simulink model "sixDOF"  (R2020b)
settings: Solver=VariableStepAuto  StartTime=0.0  StopTime=50  RelTol=1e-3
values from neighbouring files (symbols this model uses):
  A_AD = horzcat(A_i, A_ii)    [six.m]
  A_kal = [0 0 0 1 0 0 ... (first row only)    [six.m]
  B_AD = horzcat(B_i, B_ii)    [six.m]
  B_kal = [0 0 0 0 0 0 ... (first row only)    [six.m]
  C_AD = eye(6)    [six.m]
  C_D = 0.2    [Point_Mass.m]    (also in Point_mass_fancy_results.m = 0.6; point_mass_MAIN.m = 0.02; point_mass_unit_test_func.m = C_D; point_mass_verification.m)
  C_kal = eye(6)    [six.m]
  D_AD = zeros(6)    [six.m]
  D_kal = zeros(6)    [six.m]
  g = theta_dd_0*theta_d_0*cos(theta_0)*I_xy - phi_d_0*(theta_d_0)^2*sin(theta_0)*I_xy - phi_dd_0*theta_d_0*sin(theta_0)*I_xz - theta_d_0^2 * cos(theta_0)*I_xz + phi_d_0 * I_zx * theta_d_0 * cos(theta_0) + I_zy*phi_d_0^2*theta_d_0*sin(2*theta_0) + I_zz*phi_d_0 * theta_d_0 * cos(2*theta_0) + phi_d_0 * theta_d_0 * I_yx * sin(theta_0) - phi_d_0^2 * I_yy * theta_d_0 * cos(2*theta_0) + phi_d_0^2 * theta_d_0  ...(+23 chars)    [Gyro.m]    (also in Point_Mass.m = 9.81; Point_mass_fancy_results.m = 9.81; Tdt.m = cos(phi)*sin(theta)*cos(psi) + sin(phi)*sin(psi); angular_tune.m = (I_yx*I_zy - I_yy*I_zx)*(I_zx*wy_0 - I_yx*wz_0) + (I_xy*I_zx)
  I_inv = diag(I_mat)    [Propellers_tilt.m]    (also in six.m = Inertia_inv; tilt_verification.m = I_inv*0)
  I_mat = I_diag    [Propellers_tilt.m]    (also in six.m = Inertia; tilt_verification.m = 0)
  m = theta_d_0*cos(theta_0)*I_yy - theta_d_0*sin(theta_0)*I_yz + I_xx*cos(theta_0)*theta_d_0 + 2*phi_d_0*I_xy*cos(theta_0)*sin(theta_0) + 2*phi_d_0*I_xz*(cos(theta_0))^2 - theta_d_0 * I_zy * sin(theta_0) - theta_d_0*cos(theta_0)*I_zz    [Gyro.m]    (also in Point_Mass.m = 100; Point_mass_fancy_results.m = 600; point_mass_MAIN.m = 640; point_mass_unit_test_func.m = mass)
  rho = 0.991    [Point_Mass.m]    (also in Point_mass_fancy_results.m = 1.225; point_mass_MAIN.m = 1.225; point_mass_unit_test_func.m = density; point_mass_verification.m = 1.225)
  S = 4.5    [Point_Mass.m]    (also in Point_mass_fancy_results.m = 1.8; point_mass_MAIN.m = 2; point_mass_unit_test_func.m = S; point_mass_verification.m = 2)
  T = 10.5    [Point_mass_fancy_results.m]    (also in point_mass_MAIN.m; point_mass_unit_test_func.m = T; point_mass_verification.m = 1.5; six.m)
  time_delay = 0.3    [Point_mass_fancy_results.m]    (also in point_mass_MAIN.m = 3e-05; point_mass_unit_test_func.m = time_delay; point_mass_verification.m = 0.1; six.m = 0.1)
undefined symbols (not defined in the file or in its folder): Continuous, Time
libraries: pid_lib x6, ctrlSharedLib x2, simulink x2, sharedutil x1
settings Model: Creator=Jonathan van Zyl  LastModifiedBy=Jonathan van Zyl

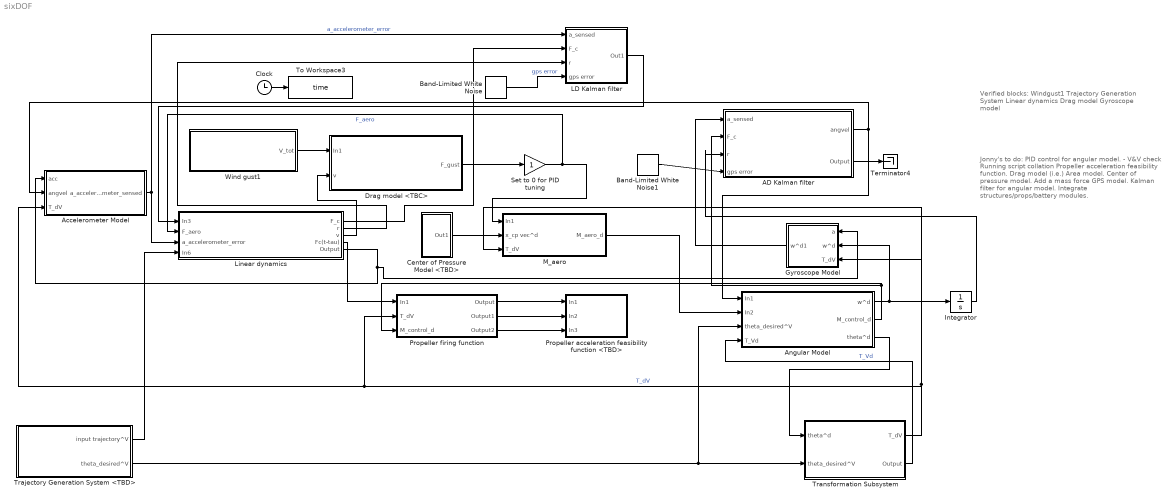
== system sixDOF ==
  note: Jonny's to do:
      | PID control for angular model. - V&V check
      | Running script collation
      | Propeller acceleration feasibility function.
      | Drag model (i.e.) Area model.
      | Center of pressure model.
      | Add a mass force
      | GPS model.
      | Kalman filter for angular model.
      | Integrate structures/props/battery modules.
  note: Verified blocks:
      | Windgust1
      | Trajectory Generation System
      | Linear dynamics
      | Drag model
      | Gyroscope model
  AD Kalman filter : Subsystem
  Accelerometer Model : Subsystem
  Angular Model : Subsystem
  Band-Limited White Noise : simulink/Sources/Band-Limited White Noise  Cov=[0.01]  Ts=0.1  seed=[23341]
  Band-Limited White Noise1 : simulink/Sources/Band-Limited White Noise  Cov=[0.01]  Ts=0.1  seed=[23341]
  Center of Pressure Model <TBD> : Subsystem
  Clock : Clock
  Drag model <TBC> : Subsystem
  Gyroscope Model : Subsystem
  Integrator : Integrator  InitialCondition=[0;0;0]
  LD Kalman filter : Subsystem
  Linear dynamics : Subsystem
  M_aero : Subsystem
  Propeller acceleration feasibility function <TBD> : Subsystem
  Propeller firing function : Subsystem
  Set to 0 for PID tuning : Gain
  Terminator4 : Terminator
  To Workspace3 : ToWorkspace  VariableName=time  SaveFormat=Structure  SampleTime=-1
      settings: Save2DSignal=2-D array (concatenate along first dimension)
  Trajectory Generation System <TBD> : Subsystem
  Transformation Subsystem : Subsystem
  Wind gust1 : Subsystem
  wires:
  Clock/1 -> To Workspace3/1
  Wind gust1/1(V_tot) -> Drag model <TBC>/1(In1)
  Drag model <TBC>/1(F_gust) -> Set to 0 for PID tuning/1
  Transformation Subsystem/1(T_dV) -> Gyroscope Model/3(T_dV), Accelerometer Model/3(T_dV), Propeller firing function/2(T_dV), M_aero/3(T_dV)  "T_dV"
  Center of Pressure Model <TBD>/1(Out1) -> M_aero/2(x_cp vec^d)
  M_aero/1(M_aero_d) -> Angular Model/2(In2)
  Transformation Subsystem/2(Output) -> Angular Model/4(T_Vd)  "T_Vd"
  Angular Model/1(w^d) -> Integrator/1, Gyroscope Model/2(w^d)
  Angular Model/2(M_control_d) -> AD Kalman filter/2(F_c), Propeller firing function/3(M_control_d)
  Angular Model/3(theta^d) -> Transformation Subsystem/1(theta^d)
  Trajectory Generation System <TBD>/2(theta_desired^V) -> Transformation Subsystem/2(theta_desired^V), Angular Model/3(theta_desired^V)
  Propeller firing function/1(Output) -> Propeller acceleration feasibility function <TBD>/1(In1)
  Propeller firing function/2(Output1) -> Propeller acceleration feasibility function <TBD>/2(In2)
  Propeller firing function/3(Output2) -> Propeller acceleration feasibility function <TBD>/3(In3)
  Band-Limited White Noise/1 -> LD Kalman filter/4(gps error)  "gps error"
  Set to 0 for PID tuning/1 -> Linear dynamics/2(F_aero), M_aero/1(In1)  "F_aero"
  Linear dynamics/5(Output) -> Gyroscope Model/1(a), Accelerometer Model/1(acc)
  LD Kalman filter/1(Out1) -> Linear dynamics/1(In3)
  Accelerometer Model/1(a_accelerometer_sensed) -> Linear dynamics/3(a_accelerometer_error), LD Kalman filter/1(a_sensed)  "a_accelerometer_error"
  Trajectory Generation System <TBD>/1(input trajectory^V) -> Linear dynamics/4(In6)
  Linear dynamics/1(F_c) -> LD Kalman filter/2(F_c)
  Linear dynamics/2(r) -> LD Kalman filter/3(r)
  Linear dynamics/3(v) -> Drag model <TBC>/2(v)
  Linear dynamics/4(Fc(t-tau)) -> Propeller firing function/1(In1)
  AD Kalman filter/1(angvel) -> Angular Model/1(In1), Accelerometer Model/2(angvel)
  Gyroscope Model/1(w^d1) -> AD Kalman filter/1(a_sensed)
  AD Kalman filter/2(Output) -> Terminator4/1
  Integrator/1 -> AD Kalman filter/3(r)
  Band-Limited White Noise1/1 -> AD Kalman filter/4(gps error)

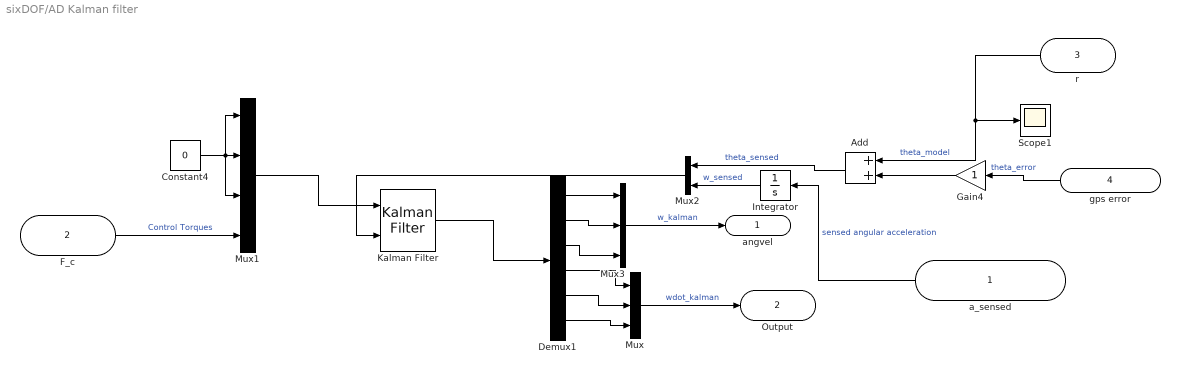
== system sixDOF/AD Kalman filter ==
  a_sensed : Inport
  F_c : Inport  Port=2
  r : Inport  Port=3
  gps error : Inport  Port=4
  Add : Sum
  Constant4 : Constant  Value=0
  Demux1 : Demux  Outputs=6
  Gain4 : Gain
  Integrator : Integrator  InitialCondition=[0;0;0]
  Kalman Filter : ctrlSharedLib/Kalman Filter  TimeDomain=Continuous-Time  UseCurrentEstimator=on  ModelSource=Individual A, B, C, D matrices  ModelSourceVariable=ss(0.95,1,1,0,1)  A=A_AD  B=B_AD  C=C_AD  D=D_AD  NumberOfStates=1  NumberOfInputs=1  NumberOfOutputs=1  InitialEstimateSource=Dialog  X0=[0;0;0;0;0;0]  P0=10  UseK=off  UseGH=off  NumberOfProcessNoiseInputs=1  G=1  TimeInvariantG=on  H=0  TimeInvariantH=on  Q=0.05  TimeInvariantQ=on  R=1  TimeInvariantR=on  N=0  TimeInvariantN=on  AddInputPort=on  AddEnablePort=off  OutputEstimatedY=off  OutputP=off  Ts=-1
  Mux : Mux  Inputs=3
  Mux1 : Mux
  Mux2 : Mux  Inputs=2
  Mux3 : Mux  Inputs=3
  Scope1 : Scope
  angvel : Outport
  Output : Outport  Port=2
  wires:
  Demux1/5 -> Mux/2
  Mux2/1 -> Kalman Filter/2
  Constant4/1 -> Mux1/3, Mux1/1, Mux1/2
  gps error/1 -> Gain4/1  "theta_error"
  r/1 -> Scope1/1, Add/1  "theta_model"
  Demux1/4 -> Mux/1
  Demux1/2 -> Mux3/2
  Mux1/1 -> Kalman Filter/1
  F_c/1 -> Mux1/4  "Control Torques"
  Demux1/1 -> Mux3/1
  Kalman Filter/1 -> Demux1/1
  Demux1/6 -> Mux/3
  Gain4/1 -> Add/2
  Demux1/3 -> Mux3/3
  Integrator/1 -> Mux2/2  "w_sensed"
  Add/1 -> Mux2/1  "theta_sensed"
  Mux3/1 -> angvel/1  "w_kalman"
  a_sensed/1 -> Integrator/1  "sensed angular acceleration"
  Mux/1 -> Output/1  "wdot_kalman"

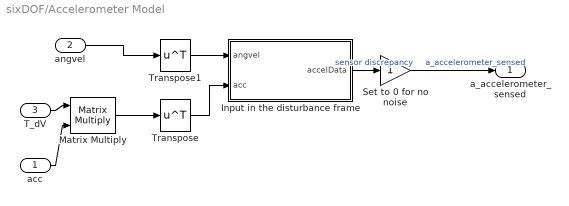
== system sixDOF/Accelerometer Model ==
  acc : Inport
  angvel : Inport  Port=2
  T_dV : Inport  Port=3
  Input in the disturbance frame : MATLAB Function  TreatAsAtomicUnit=on
  Matrix Multiply : Product  Multiplication=Matrix(*)
  Set to 0 for no noise : Gain
  Transpose : Math  Operator=transpose  SaturateOnIntegerOverflow=on
  Transpose1 : Math  Operator=transpose  SaturateOnIntegerOverflow=on
  a_accelerometer_sensed : Outport
  wires:
  Input in the disturbance frame/1(accelData) -> Set to 0 for no noise/1  "sensor discrepancy"
  acc/1 -> Matrix Multiply/2
  angvel/1 -> Transpose1/1
  Set to 0 for no noise/1 -> a_accelerometer_sensed/1  "a_accelerometer_sensed"
  Matrix Multiply/1 -> Transpose/1
  T_dV/1 -> Matrix Multiply/1
  Transpose/1 -> Input in the disturbance frame/2(acc)
  Transpose1/1 -> Input in the disturbance frame/1(angvel)

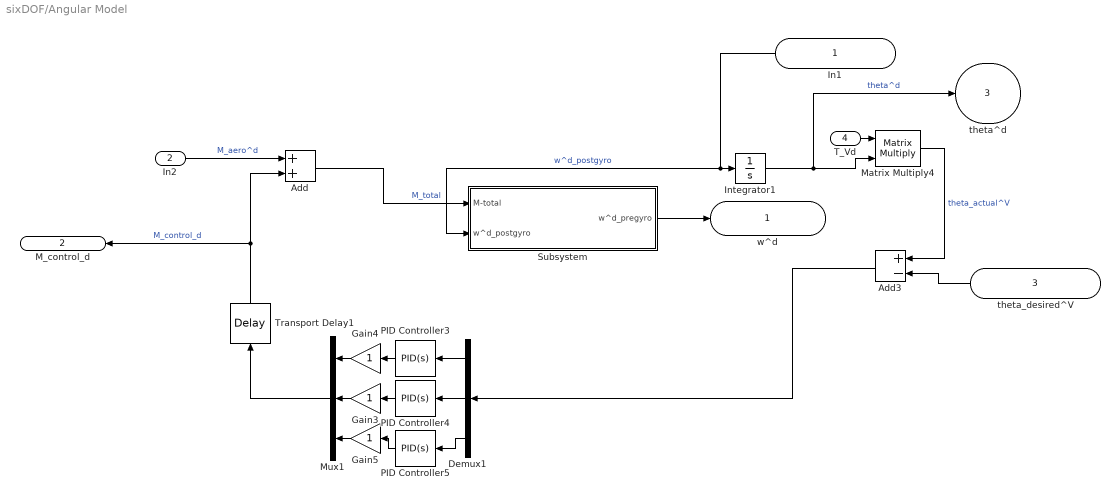
== system sixDOF/Angular Model ==
  In1 : Inport
  In2 : Inport  Port=2
  theta_desired^V : Inport  Port=3
  T_Vd : Inport  Port=4
  Add : Sum
  Add3 : Sum  Inputs=+-
  Demux1 : Demux  Outputs=3
  Gain3 : Gain
  Gain4 : Gain
  Gain5 : Gain
  Integrator1 : Integrator  InitialCondition=[0;0;0]
  Matrix Multiply4 : Product  Multiplication=Matrix(*)
  Mux1 : Mux  Inputs=3
  PID Controller3 : pid_lib/PID Controller  Controller=PID  Form=Parallel  TimeDomain=Continuous-time  UseExternalTs=off  SampleTime=-1  IntegratorMethod=Forward Euler  FilterMethod=Forward Euler  ControllerParametersSource=internal  P=1  I=1  D=0  UseFilter=on  N=100  TunerSelectOption=Transfer Function Based (PID Tuner App)  InitialConditionSource=internal  InitialConditionForIntegrator=0  InitialConditionForFilter=0  DifferentiatorICPrevScaledInput=0  ExternalReset=none  TrackingMode=off  Kt=1  LimitOutput=off  SatLimitsSource=internal  UpperSaturationLimit=inf  LowerSaturationLimit=-inf  LinearizeAsGain=on  AntiWindupMode=none  Kb=1  POutMin=[]  POutMax=[]  IOutMin=[]  IOutMax=[]  DOutMin=[]  DOutMax=[]  NOutMin=[]  NOutMax=[]  SumOutMin=[]  SumOutMax=[]  SaturationOutMin=[]  SaturationOutMax=[]  PParamMin=[]  PParamMax=[]  IParamMin=[]  IParamMax=[]  DParamMin=[]  DParamMax=[]  NParamMin=[]  NParamMax=[]  KbParamMin=[]  KbParamMax=[]  KtParamMin=[]  KtParamMax=[]  KbOutMin=[]  KbOutMax=[]  KtOutMin=[]  KtOutMax=[]  IntegratorOutMin=[]  IntegratorOutMax=[]  FilterOutMin=[]  FilterOutMax=[]  SumI1OutMin=[]  SumI1OutMax=[]  SumI2OutMin=[]  SumI2OutMax=[]  SumI3OutMin=[]  SumI3OutMax=[]  SumI4OutMin=[]  SumI4OutMax=[]  SumDOutMin=[]  SumDOutMax=[]  DifferentiatorOutMin=[]  DifferentiatorOutMax=[]  FilterDiffOutCoefMin=[]  FilterDiffOutCoefMax=[]  ReciprocalOutMin=[]  ReciprocalOutMax=[]  SumDenOutMin=[]  SumDenOutMax=[]  SumNumOutMin=[]  SumNumOutMax=[]  DivideOutMin=[]  DivideOutMax=[]  UdiffTsProdOutMin=[]  UdiffTsProdOutMax=[]  NTsProdOutMin=[]  NTsProdOutMax=[]  UintegralTsProdOutMin=[]  UintegralTsProdOutMax=[]  UngainTsProdOutMin=[]  UngainTsProdOutMax=[]  IntegratorContinuousStateAttributes=''  IntegratorStateMustResolveToSignalObject=off  IntegratorRTWStateStorageClass=Auto  FilterContinuousStateAttributes=''  FilterStateMustResolveToSignalObject=off  FilterRTWStateStorageClass=Auto  ParallelPVariant=InternalParameters  IdealPVariant=Disabled  IVariant=InternalParameters  DVariant=InternalParameters  IntegratorVariant=Continuous  SatVariant=Disabled  AWVariant=Passthrough  PCopyVariant=Disabled  TRVariant=Disabled  FdbkBlocksVariant=Forward  IdealPFdbkVariant=Disabled  SatFdbkVariant=Disabled  DerivativeFilterVariant=ContFilter  NVariant=InternalParameters  NCopyVariant=Disabled  FilterICVariant=InternalICsFilter  IntegratorICVariant=InternalICs  ExternalResetVariant=Disabled  TRSumVariant=Passthrough  SumFdbkVariant=Disabled  SumVariant=Sum_PID  TsampFilterVariant=InternalTs  TsampNgainVariant=Passthrough  TsampIntegralVariant=Passthrough  ExternalSaturationOutDataTypeStr=Inherit: Same as second input
  PID Controller4 : pid_lib/PID Controller  Controller=PID  Form=Parallel  TimeDomain=Continuous-time  UseExternalTs=off  SampleTime=-1  IntegratorMethod=Forward Euler  FilterMethod=Forward Euler  ControllerParametersSource=internal  P=1  I=1  D=0  UseFilter=on  N=100  TunerSelectOption=Transfer Function Based (PID Tuner App)  InitialConditionSource=internal  InitialConditionForIntegrator=0  InitialConditionForFilter=0  DifferentiatorICPrevScaledInput=0  ExternalReset=none  TrackingMode=off  Kt=1  LimitOutput=off  SatLimitsSource=internal  UpperSaturationLimit=inf  LowerSaturationLimit=-inf  LinearizeAsGain=on  AntiWindupMode=none  Kb=1  POutMin=[]  POutMax=[]  IOutMin=[]  IOutMax=[]  DOutMin=[]  DOutMax=[]  NOutMin=[]  NOutMax=[]  SumOutMin=[]  SumOutMax=[]  SaturationOutMin=[]  SaturationOutMax=[]  PParamMin=[]  PParamMax=[]  IParamMin=[]  IParamMax=[]  DParamMin=[]  DParamMax=[]  NParamMin=[]  NParamMax=[]  KbParamMin=[]  KbParamMax=[]  KtParamMin=[]  KtParamMax=[]  KbOutMin=[]  KbOutMax=[]  KtOutMin=[]  KtOutMax=[]  IntegratorOutMin=[]  IntegratorOutMax=[]  FilterOutMin=[]  FilterOutMax=[]  SumI1OutMin=[]  SumI1OutMax=[]  SumI2OutMin=[]  SumI2OutMax=[]  SumI3OutMin=[]  SumI3OutMax=[]  SumI4OutMin=[]  SumI4OutMax=[]  SumDOutMin=[]  SumDOutMax=[]  DifferentiatorOutMin=[]  DifferentiatorOutMax=[]  FilterDiffOutCoefMin=[]  FilterDiffOutCoefMax=[]  ReciprocalOutMin=[]  ReciprocalOutMax=[]  SumDenOutMin=[]  SumDenOutMax=[]  SumNumOutMin=[]  SumNumOutMax=[]  DivideOutMin=[]  DivideOutMax=[]  UdiffTsProdOutMin=[]  UdiffTsProdOutMax=[]  NTsProdOutMin=[]  NTsProdOutMax=[]  UintegralTsProdOutMin=[]  UintegralTsProdOutMax=[]  UngainTsProdOutMin=[]  UngainTsProdOutMax=[]  IntegratorContinuousStateAttributes=''  IntegratorStateMustResolveToSignalObject=off  IntegratorRTWStateStorageClass=Auto  FilterContinuousStateAttributes=''  FilterStateMustResolveToSignalObject=off  FilterRTWStateStorageClass=Auto  ParallelPVariant=InternalParameters  IdealPVariant=Disabled  IVariant=InternalParameters  DVariant=InternalParameters  IntegratorVariant=Continuous  SatVariant=Disabled  AWVariant=Passthrough  PCopyVariant=Disabled  TRVariant=Disabled  FdbkBlocksVariant=Forward  IdealPFdbkVariant=Disabled  SatFdbkVariant=Disabled  DerivativeFilterVariant=ContFilter  NVariant=InternalParameters  NCopyVariant=Disabled  FilterICVariant=InternalICsFilter  IntegratorICVariant=InternalICs  ExternalResetVariant=Disabled  TRSumVariant=Passthrough  SumFdbkVariant=Disabled  SumVariant=Sum_PID  TsampFilterVariant=InternalTs  TsampNgainVariant=Passthrough  TsampIntegralVariant=Passthrough  ExternalSaturationOutDataTypeStr=Inherit: Same as second input
  PID Controller5 : pid_lib/PID Controller  Controller=PID  Form=Parallel  TimeDomain=Continuous-time  UseExternalTs=off  SampleTime=-1  IntegratorMethod=Forward Euler  FilterMethod=Forward Euler  ControllerParametersSource=internal  P=1  I=1  D=0  UseFilter=on  N=100  TunerSelectOption=Transfer Function Based (PID Tuner App)  InitialConditionSource=internal  InitialConditionForIntegrator=0  InitialConditionForFilter=0  DifferentiatorICPrevScaledInput=0  ExternalReset=none  TrackingMode=off  Kt=1  LimitOutput=off  SatLimitsSource=internal  UpperSaturationLimit=inf  LowerSaturationLimit=-inf  LinearizeAsGain=on  AntiWindupMode=none  Kb=1  POutMin=[]  POutMax=[]  IOutMin=[]  IOutMax=[]  DOutMin=[]  DOutMax=[]  NOutMin=[]  NOutMax=[]  SumOutMin=[]  SumOutMax=[]  SaturationOutMin=[]  SaturationOutMax=[]  PParamMin=[]  PParamMax=[]  IParamMin=[]  IParamMax=[]  DParamMin=[]  DParamMax=[]  NParamMin=[]  NParamMax=[]  KbParamMin=[]  KbParamMax=[]  KtParamMin=[]  KtParamMax=[]  KbOutMin=[]  KbOutMax=[]  KtOutMin=[]  KtOutMax=[]  IntegratorOutMin=[]  IntegratorOutMax=[]  FilterOutMin=[]  FilterOutMax=[]  SumI1OutMin=[]  SumI1OutMax=[]  SumI2OutMin=[]  SumI2OutMax=[]  SumI3OutMin=[]  SumI3OutMax=[]  SumI4OutMin=[]  SumI4OutMax=[]  SumDOutMin=[]  SumDOutMax=[]  DifferentiatorOutMin=[]  DifferentiatorOutMax=[]  FilterDiffOutCoefMin=[]  FilterDiffOutCoefMax=[]  ReciprocalOutMin=[]  ReciprocalOutMax=[]  SumDenOutMin=[]  SumDenOutMax=[]  SumNumOutMin=[]  SumNumOutMax=[]  DivideOutMin=[]  DivideOutMax=[]  UdiffTsProdOutMin=[]  UdiffTsProdOutMax=[]  NTsProdOutMin=[]  NTsProdOutMax=[]  UintegralTsProdOutMin=[]  UintegralTsProdOutMax=[]  UngainTsProdOutMin=[]  UngainTsProdOutMax=[]  IntegratorContinuousStateAttributes=''  IntegratorStateMustResolveToSignalObject=off  IntegratorRTWStateStorageClass=Auto  FilterContinuousStateAttributes=''  FilterStateMustResolveToSignalObject=off  FilterRTWStateStorageClass=Auto  ParallelPVariant=InternalParameters  IdealPVariant=Disabled  IVariant=InternalParameters  DVariant=InternalParameters  IntegratorVariant=Continuous  SatVariant=Disabled  AWVariant=Passthrough  PCopyVariant=Disabled  TRVariant=Disabled  FdbkBlocksVariant=Forward  IdealPFdbkVariant=Disabled  SatFdbkVariant=Disabled  DerivativeFilterVariant=ContFilter  NVariant=InternalParameters  NCopyVariant=Disabled  FilterICVariant=InternalICsFilter  IntegratorICVariant=InternalICs  ExternalResetVariant=Disabled  TRSumVariant=Passthrough  SumFdbkVariant=Disabled  SumVariant=Sum_PID  TsampFilterVariant=InternalTs  TsampNgainVariant=Passthrough  TsampIntegralVariant=Passthrough  ExternalSaturationOutDataTypeStr=Inherit: Same as second input
  Subsystem : Subsystem
  Transport Delay1 : TransportDelay  DelayTime=time_delay  TransDelayFeedthrough=on
  w^d : Outport
  M_control_d : Outport  Port=2
  theta^d : Outport  Port=3
  wires:
  Matrix Multiply4/1 -> Add3/1  "theta_actual^V"
  Demux1/1 -> PID Controller3/1
  In2/1 -> Add/1  "M_aero^d"
  PID Controller3/1 -> Gain4/1
  Mux1/1 -> Transport Delay1/1
  Add3/1 -> Demux1/1
  In1/1 -> Subsystem/2(w^d_postgyro), Integrator1/1  "w^d_postgyro"
  Demux1/3 -> PID Controller5/1
  Transport Delay1/1 -> Add/2, M_control_d/1  "M_control_d"
  PID Controller5/1 -> Gain5/1
  Demux1/2 -> PID Controller4/1
  Gain3/1 -> Mux1/2
  PID Controller4/1 -> Gain3/1
  Integrator1/1 -> theta^d/1, Matrix Multiply4/2  "theta^d"
  Gain5/1 -> Mux1/3
  theta_desired^V/1 -> Add3/2
  Gain4/1 -> Mux1/1
  T_Vd/1 -> Matrix Multiply4/1
  Add/1 -> Subsystem/1(M-total)  "M_total"
  Subsystem/1(w^d_pregyro) -> w^d/1

== system sixDOF/Center of Pressure Model <TBD> ==
  Constant1 : Constant  Value=[0.1;0.2; 0.05]
  Out1 : Outport
  wires:
  Constant1/1 -> Out1/1  "x_cp"

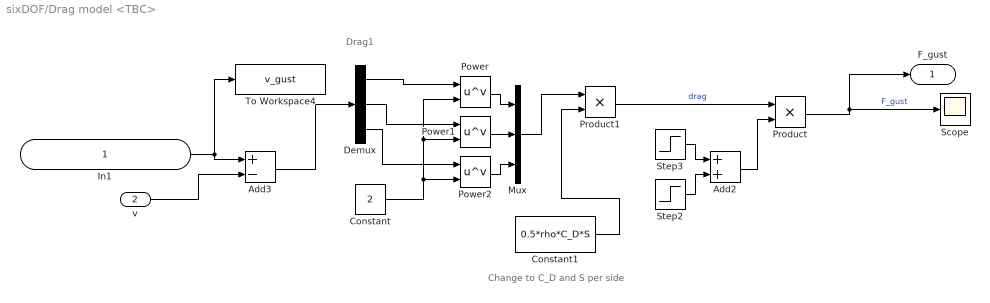
== system sixDOF/Drag model <TBC> ==
  note: Drag1
  note: Change to C_D and S per side
  In1 : Inport
  v : Inport  Port=2
  Add2 : Sum
  Add3 : Sum  Inputs=+-
  Constant : Constant  Value=2
  Constant1 : Constant  Value=0.5*rho*C_D*S
  Demux : Demux  Outputs=3
  Mux : Mux  Inputs=3
  Power : Math  Operator=pow  SaturateOnIntegerOverflow=on
  Power1 : Math  Operator=pow  SaturateOnIntegerOverflow=on
  Power2 : Math  Operator=pow  SaturateOnIntegerOverflow=on
  Product : Product
  Product1 : Product
  Scope : Scope
  Step2 : Step  Time=0  SampleTime=0
  Step3 : Step  Time=10.5  After=-1  SampleTime=0
  To Workspace4 : ToWorkspace  VariableName=v_gust  SaveFormat=Timeseries  SampleTime=-1
  F_gust : Outport
  wires:
  Add2/1 -> Product/2
  Step2/1 -> Add2/2
  v/1 -> Add3/2
  Product/1 -> F_gust/1, Scope/1  "F_gust"
  Step3/1 -> Add2/1
  In1/1 -> Add3/1, To Workspace4/1
  Mux/1 -> Product1/1
  Power2/1 -> Mux/3
  Power1/1 -> Mux/2
  Demux/3 -> Power2/1
  Demux/2 -> Power1/1
  Demux/1 -> Power/1
  Power/1 -> Mux/1
  Add3/1 -> Demux/1
  Constant/1 -> Power2/2, Power1/2, Power/2
  Product1/1 -> Product/1  "drag"
  Constant1/1 -> Product1/2

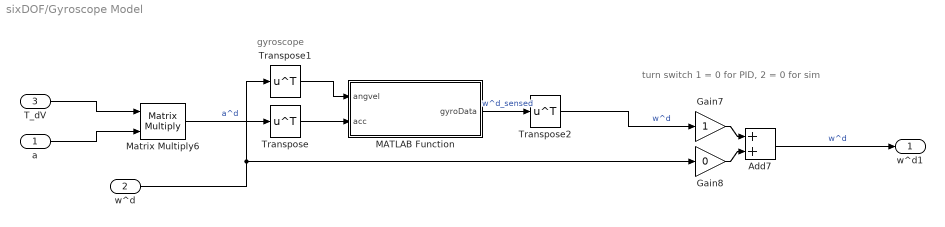
== system sixDOF/Gyroscope Model ==
  note: gyroscope
  note: turn switch 1 = 0 for PID, 2 = 0 for sim
  a : Inport
  w^d : Inport  Port=2
  T_dV : Inport  Port=3
  Add7 : Sum
  Gain7 : Gain
  Gain8 : Gain  Gain=0
  MATLAB Function : MATLAB Function  TreatAsAtomicUnit=on
  Matrix Multiply6 : Product  Multiplication=Matrix(*)
  Transpose : Math  Operator=transpose  SaturateOnIntegerOverflow=on
  Transpose1 : Math  Operator=transpose  SaturateOnIntegerOverflow=on
  Transpose2 : Math  Operator=transpose  SaturateOnIntegerOverflow=on
  w^d1 : Outport
  wires:
  a/1 -> Matrix Multiply6/2
  Matrix Multiply6/1 -> Transpose/1  "a^d"
  T_dV/1 -> Matrix Multiply6/1
  Add7/1 -> w^d1/1  "w^d"
  Gain8/1 -> Add7/2
  Gain7/1 -> Add7/1
  Transpose2/1 -> Gain7/1  "w^d"
  w^d/1 -> Transpose1/1, Gain8/1
  Transpose1/1 -> MATLAB Function/1(angvel)
  MATLAB Function/1(gyroData) -> Transpose2/1  "w^d_sensed"
  Transpose/1 -> MATLAB Function/2(acc)

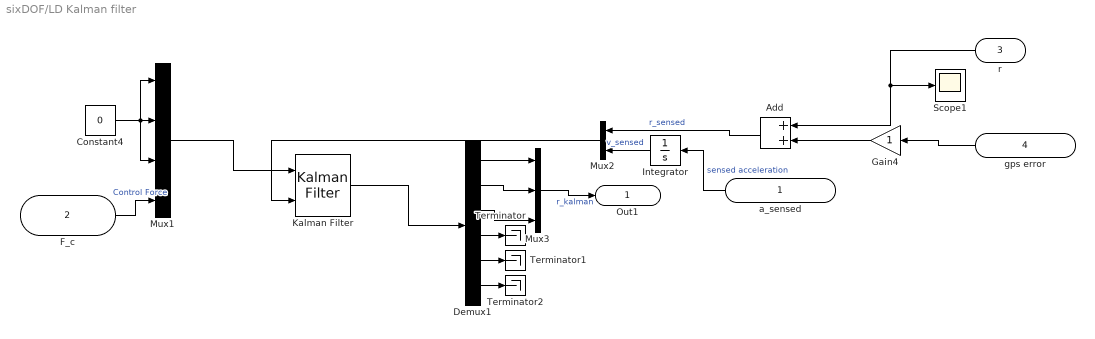
== system sixDOF/LD Kalman filter ==
  a_sensed : Inport
  F_c : Inport  Port=2
  r : Inport  Port=3
  gps error : Inport  Port=4
  Add : Sum
  Constant4 : Constant  Value=0
  Demux1 : Demux  Outputs=6
  Gain4 : Gain
  Integrator : Integrator  InitialCondition=[0;0;0]
  Kalman Filter : ctrlSharedLib/Kalman Filter  TimeDomain=Continuous-Time  UseCurrentEstimator=on  ModelSource=Individual A, B, C, D matrices  ModelSourceVariable=ss(0.95,1,1,0,1)  A=A_kal  B=B_kal  C=C_kal  D=D_kal  NumberOfStates=1  NumberOfInputs=1  NumberOfOutputs=1  InitialEstimateSource=Dialog  X0=[0;0;0;0;0;0]  P0=10  UseK=off  UseGH=off  NumberOfProcessNoiseInputs=1  G=1  TimeInvariantG=on  H=0  TimeInvariantH=on  Q=0.05  TimeInvariantQ=on  R=1  TimeInvariantR=on  N=0  TimeInvariantN=on  AddInputPort=on  AddEnablePort=off  OutputEstimatedY=off  OutputP=off  Ts=-1
  Mux1 : Mux
  Mux2 : Mux  Inputs=2
  Mux3 : Mux  Inputs=3
  Scope1 : Scope
  Terminator : Terminator
  Terminator1 : Terminator
  Terminator2 : Terminator
  Out1 : Outport
  wires:
  Demux1/5 -> Terminator1/1
  Mux2/1 -> Kalman Filter/2
  Constant4/1 -> Mux1/3, Mux1/1, Mux1/2
  gps error/1 -> Gain4/1
  r/1 -> Scope1/1, Add/1
  Demux1/4 -> Terminator/1
  Demux1/2 -> Mux3/2
  Mux1/1 -> Kalman Filter/1
  F_c/1 -> Mux1/4  "Control Force"
  Demux1/1 -> Mux3/1
  Kalman Filter/1 -> Demux1/1
  Demux1/6 -> Terminator2/1
  Gain4/1 -> Add/2
  Demux1/3 -> Mux3/3
  Integrator/1 -> Mux2/2  "v_sensed"
  Add/1 -> Mux2/1  "r_sensed"
  Mux3/1 -> Out1/1  "r_kalman"
  a_sensed/1 -> Integrator/1  "sensed acceleration"

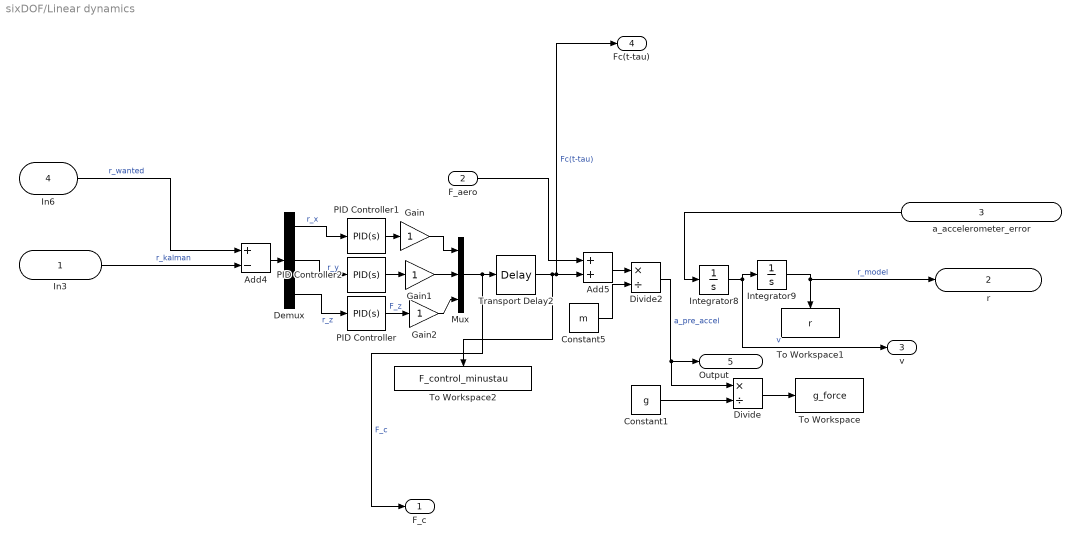
== system sixDOF/Linear dynamics ==
  In3 : Inport
  F_aero : Inport  Port=2
  a_accelerometer_error : Inport  Port=3
  In6 : Inport  Port=4
  Add4 : Sum  Inputs=+-
  Add5 : Sum
  Constant1 : Constant  Value=g
  Constant5 : Constant  Value=m
  Demux : Demux  Outputs=3
  Divide : Product  Inputs=*/
  Divide2 : Product  Inputs=*/
  Gain : Gain
  Gain1 : Gain
  Gain2 : Gain
  Integrator8 : Integrator  InitialCondition=[0;0;0]
  Integrator9 : Integrator  InitialCondition=[0;0;0]
  Mux : Mux  Inputs=3
  PID Controller : pid_lib/PID Controller  Controller=PID  Form=Parallel  TimeDomain=Continuous-time  UseExternalTs=off  SampleTime=-1  IntegratorMethod=Forward Euler  FilterMethod=Forward Euler  ControllerParametersSource=internal  P=86.974466686756  I=2.5080869601386  D=635.831408940251  UseFilter=on  N=114.28279760416  TunerSelectOption=Transfer Function Based (PID Tuner App)  InitialConditionSource=internal  InitialConditionForIntegrator=0  InitialConditionForFilter=0  DifferentiatorICPrevScaledInput=0  ExternalReset=none  TrackingMode=off  Kt=1  LimitOutput=off  SatLimitsSource=internal  UpperSaturationLimit=inf  LowerSaturationLimit=-inf  LinearizeAsGain=on  AntiWindupMode=none  Kb=1  POutMin=[]  POutMax=[]  IOutMin=[]  IOutMax=[]  DOutMin=[]  DOutMax=[]  NOutMin=[]  NOutMax=[]  SumOutMin=[]  SumOutMax=[]  SaturationOutMin=[]  SaturationOutMax=[]  PParamMin=[]  PParamMax=[]  IParamMin=[]  IParamMax=[]  DParamMin=[]  DParamMax=[]  NParamMin=[]  NParamMax=[]  KbParamMin=[]  KbParamMax=[]  KtParamMin=[]  KtParamMax=[]  KbOutMin=[]  KbOutMax=[]  KtOutMin=[]  KtOutMax=[]  IntegratorOutMin=[]  IntegratorOutMax=[]  FilterOutMin=[]  FilterOutMax=[]  SumI1OutMin=[]  SumI1OutMax=[]  SumI2OutMin=[]  SumI2OutMax=[]  SumI3OutMin=[]  SumI3OutMax=[]  SumI4OutMin=[]  SumI4OutMax=[]  SumDOutMin=[]  SumDOutMax=[]  DifferentiatorOutMin=[]  DifferentiatorOutMax=[]  FilterDiffOutCoefMin=[]  FilterDiffOutCoefMax=[]  ReciprocalOutMin=[]  ReciprocalOutMax=[]  SumDenOutMin=[]  SumDenOutMax=[]  SumNumOutMin=[]  SumNumOutMax=[]  DivideOutMin=[]  DivideOutMax=[]  UdiffTsProdOutMin=[]  UdiffTsProdOutMax=[]  NTsProdOutMin=[]  NTsProdOutMax=[]  UintegralTsProdOutMin=[]  UintegralTsProdOutMax=[]  UngainTsProdOutMin=[]  UngainTsProdOutMax=[]  IntegratorContinuousStateAttributes=''  IntegratorStateMustResolveToSignalObject=off  IntegratorRTWStateStorageClass=Auto  FilterContinuousStateAttributes=''  FilterStateMustResolveToSignalObject=off  FilterRTWStateStorageClass=Auto  ParallelPVariant=InternalParameters  IdealPVariant=Disabled  IVariant=InternalParameters  DVariant=InternalParameters  IntegratorVariant=Continuous  SatVariant=Disabled  AWVariant=Passthrough  PCopyVariant=Disabled  TRVariant=Disabled  FdbkBlocksVariant=Forward  IdealPFdbkVariant=Disabled  SatFdbkVariant=Disabled  DerivativeFilterVariant=ContFilter  NVariant=InternalParameters  NCopyVariant=Disabled  FilterICVariant=InternalICsFilter  IntegratorICVariant=InternalICs  ExternalResetVariant=Disabled  TRSumVariant=Passthrough  SumFdbkVariant=Disabled  SumVariant=Sum_PID  TsampFilterVariant=InternalTs  TsampNgainVariant=Passthrough  TsampIntegralVariant=Passthrough  ExternalSaturationOutDataTypeStr=Inherit: Same as second input
  PID Controller1 : pid_lib/PID Controller  Controller=PID  Form=Parallel  TimeDomain=Continuous-time  UseExternalTs=off  SampleTime=-1  IntegratorMethod=Forward Euler  FilterMethod=Forward Euler  ControllerParametersSource=internal  P=86.974466686756  I=2.5080869601386  D=635.831408940251  UseFilter=on  N=114.28279760416  TunerSelectOption=Transfer Function Based (PID Tuner App)  InitialConditionSource=internal  InitialConditionForIntegrator=0  InitialConditionForFilter=0  DifferentiatorICPrevScaledInput=0  ExternalReset=none  TrackingMode=off  Kt=1  LimitOutput=off  SatLimitsSource=internal  UpperSaturationLimit=inf  LowerSaturationLimit=-inf  LinearizeAsGain=on  AntiWindupMode=none  Kb=1  POutMin=[]  POutMax=[]  IOutMin=[]  IOutMax=[]  DOutMin=[]  DOutMax=[]  NOutMin=[]  NOutMax=[]  SumOutMin=[]  SumOutMax=[]  SaturationOutMin=[]  SaturationOutMax=[]  PParamMin=[]  PParamMax=[]  IParamMin=[]  IParamMax=[]  DParamMin=[]  DParamMax=[]  NParamMin=[]  NParamMax=[]  KbParamMin=[]  KbParamMax=[]  KtParamMin=[]  KtParamMax=[]  KbOutMin=[]  KbOutMax=[]  KtOutMin=[]  KtOutMax=[]  IntegratorOutMin=[]  IntegratorOutMax=[]  FilterOutMin=[]  FilterOutMax=[]  SumI1OutMin=[]  SumI1OutMax=[]  SumI2OutMin=[]  SumI2OutMax=[]  SumI3OutMin=[]  SumI3OutMax=[]  SumI4OutMin=[]  SumI4OutMax=[]  SumDOutMin=[]  SumDOutMax=[]  DifferentiatorOutMin=[]  DifferentiatorOutMax=[]  FilterDiffOutCoefMin=[]  FilterDiffOutCoefMax=[]  ReciprocalOutMin=[]  ReciprocalOutMax=[]  SumDenOutMin=[]  SumDenOutMax=[]  SumNumOutMin=[]  SumNumOutMax=[]  DivideOutMin=[]  DivideOutMax=[]  UdiffTsProdOutMin=[]  UdiffTsProdOutMax=[]  NTsProdOutMin=[]  NTsProdOutMax=[]  UintegralTsProdOutMin=[]  UintegralTsProdOutMax=[]  UngainTsProdOutMin=[]  UngainTsProdOutMax=[]  IntegratorContinuousStateAttributes=''  IntegratorStateMustResolveToSignalObject=off  IntegratorRTWStateStorageClass=Auto  FilterContinuousStateAttributes=''  FilterStateMustResolveToSignalObject=off  FilterRTWStateStorageClass=Auto  ParallelPVariant=InternalParameters  IdealPVariant=Disabled  IVariant=InternalParameters  DVariant=InternalParameters  IntegratorVariant=Continuous  SatVariant=Disabled  AWVariant=Passthrough  PCopyVariant=Disabled  TRVariant=Disabled  FdbkBlocksVariant=Forward  IdealPFdbkVariant=Disabled  SatFdbkVariant=Disabled  DerivativeFilterVariant=ContFilter  NVariant=InternalParameters  NCopyVariant=Disabled  FilterICVariant=InternalICsFilter  IntegratorICVariant=InternalICs  ExternalResetVariant=Disabled  TRSumVariant=Passthrough  SumFdbkVariant=Disabled  SumVariant=Sum_PID  TsampFilterVariant=InternalTs  TsampNgainVariant=Passthrough  TsampIntegralVariant=Passthrough  ExternalSaturationOutDataTypeStr=Inherit: Same as second input
  PID Controller2 : pid_lib/PID Controller  Controller=PID  Form=Parallel  TimeDomain=Continuous-time  UseExternalTs=off  SampleTime=-1  IntegratorMethod=Forward Euler  FilterMethod=Forward Euler  ControllerParametersSource=internal  P=86.974466686756  I=2.5080869601386  D=635.831408940251  UseFilter=on  N=114.28279760416  TunerSelectOption=Transfer Function Based (PID Tuner App)  InitialConditionSource=internal  InitialConditionForIntegrator=0  InitialConditionForFilter=0  DifferentiatorICPrevScaledInput=0  ExternalReset=none  TrackingMode=off  Kt=1  LimitOutput=off  SatLimitsSource=internal  UpperSaturationLimit=inf  LowerSaturationLimit=-inf  LinearizeAsGain=on  AntiWindupMode=none  Kb=1  POutMin=[]  POutMax=[]  IOutMin=[]  IOutMax=[]  DOutMin=[]  DOutMax=[]  NOutMin=[]  NOutMax=[]  SumOutMin=[]  SumOutMax=[]  SaturationOutMin=[]  SaturationOutMax=[]  PParamMin=[]  PParamMax=[]  IParamMin=[]  IParamMax=[]  DParamMin=[]  DParamMax=[]  NParamMin=[]  NParamMax=[]  KbParamMin=[]  KbParamMax=[]  KtParamMin=[]  KtParamMax=[]  KbOutMin=[]  KbOutMax=[]  KtOutMin=[]  KtOutMax=[]  IntegratorOutMin=[]  IntegratorOutMax=[]  FilterOutMin=[]  FilterOutMax=[]  SumI1OutMin=[]  SumI1OutMax=[]  SumI2OutMin=[]  SumI2OutMax=[]  SumI3OutMin=[]  SumI3OutMax=[]  SumI4OutMin=[]  SumI4OutMax=[]  SumDOutMin=[]  SumDOutMax=[]  DifferentiatorOutMin=[]  DifferentiatorOutMax=[]  FilterDiffOutCoefMin=[]  FilterDiffOutCoefMax=[]  ReciprocalOutMin=[]  ReciprocalOutMax=[]  SumDenOutMin=[]  SumDenOutMax=[]  SumNumOutMin=[]  SumNumOutMax=[]  DivideOutMin=[]  DivideOutMax=[]  UdiffTsProdOutMin=[]  UdiffTsProdOutMax=[]  NTsProdOutMin=[]  NTsProdOutMax=[]  UintegralTsProdOutMin=[]  UintegralTsProdOutMax=[]  UngainTsProdOutMin=[]  UngainTsProdOutMax=[]  IntegratorContinuousStateAttributes=''  IntegratorStateMustResolveToSignalObject=off  IntegratorRTWStateStorageClass=Auto  FilterContinuousStateAttributes=''  FilterStateMustResolveToSignalObject=off  FilterRTWStateStorageClass=Auto  ParallelPVariant=InternalParameters  IdealPVariant=Disabled  IVariant=InternalParameters  DVariant=InternalParameters  IntegratorVariant=Continuous  SatVariant=Disabled  AWVariant=Passthrough  PCopyVariant=Disabled  TRVariant=Disabled  FdbkBlocksVariant=Forward  IdealPFdbkVariant=Disabled  SatFdbkVariant=Disabled  DerivativeFilterVariant=ContFilter  NVariant=InternalParameters  NCopyVariant=Disabled  FilterICVariant=InternalICsFilter  IntegratorICVariant=InternalICs  ExternalResetVariant=Disabled  TRSumVariant=Passthrough  SumFdbkVariant=Disabled  SumVariant=Sum_PID  TsampFilterVariant=InternalTs  TsampNgainVariant=Passthrough  TsampIntegralVariant=Passthrough  ExternalSaturationOutDataTypeStr=Inherit: Same as second input
  To Workspace : ToWorkspace  VariableName=g_force  SaveFormat=Timeseries  SampleTime=-1
      settings: Save2DSignal=2-D array (concatenate along first dimension)
  To Workspace1 : ToWorkspace  VariableName=r  SaveFormat=Timeseries  SampleTime=-1
  To Workspace2 : ToWorkspace  VariableName=F_control_minustau  SaveFormat=Timeseries  SampleTime=-1
  Transport Delay2 : TransportDelay  DelayTime=time_delay  TransDelayFeedthrough=on
  F_c : Outport
  r : Outport  Port=2
  v : Outport  Port=3
  Fc(t-tau) : Outport  Port=4
  Output : Outport  Port=5
  wires:
  Demux/2 -> PID Controller2/1  "r_y"
  Add5/1 -> Divide2/1
  PID Controller/1 -> Gain2/1  "F_z"
  Constant1/1 -> Divide/2
  Add4/1 -> Demux/1
  Transport Delay2/1 -> Fc(t-tau)/1, Add5/2, To Workspace2/1  "Fc(t-tau)"
  Gain2/1 -> Mux/3
  Demux/3 -> PID Controller/1  "r_z"
  In6/1 -> Add4/1  "r_wanted"
  PID Controller2/1 -> Gain1/1
  Integrator9/1 -> r/1, To Workspace1/1  "r_model"
  Divide/1 -> To Workspace/1
  F_aero/1 -> Add5/1
  Constant5/1 -> Divide2/2
  Demux/1 -> PID Controller1/1  "r_x"
  Mux/1 -> F_c/1, Transport Delay2/1  "F_c"
  Gain/1 -> Mux/1
  PID Controller1/1 -> Gain/1
  In3/1 -> Add4/2  "r_kalman"
  Integrator8/1 -> v/1, Integrator9/1  "v"
  Gain1/1 -> Mux/2
  Divide2/1 -> Divide/1, Output/1  "a_pre_accel"
  a_accelerometer_error/1 -> Integrator8/1

== system sixDOF/M_aero ==
  In1 : Inport
  x_cp vec^d : Inport  Port=2
  T_dV : Inport  Port=3
  Matrix Multiply : Product  Multiplication=Matrix(*)
  Matrix Multiply1 : Product  Multiplication=Matrix(*)
  M_aero_d : Outport
  wires:
  Matrix Multiply/1 -> Matrix Multiply1/2  "F_dis^d"
  x_cp vec^d/1 -> Matrix Multiply1/1  "x_cp"
  T_dV/1 -> Matrix Multiply/1
  In1/1 -> Matrix Multiply/2  "F_gust"
  Matrix Multiply1/1 -> M_aero_d/1  "M_aero_d"

== system sixDOF/Propeller acceleration feasibility function <TBD> ==
  In1 : Inport
  In2 : Inport  Port=2
  In3 : Inport  Port=3
  Terminator4 : Terminator
  Terminator5 : Terminator
  Terminator6 : Terminator
  wires:
  In1/1 -> Terminator4/1
  In2/1 -> Terminator5/1
  In3/1 -> Terminator6/1

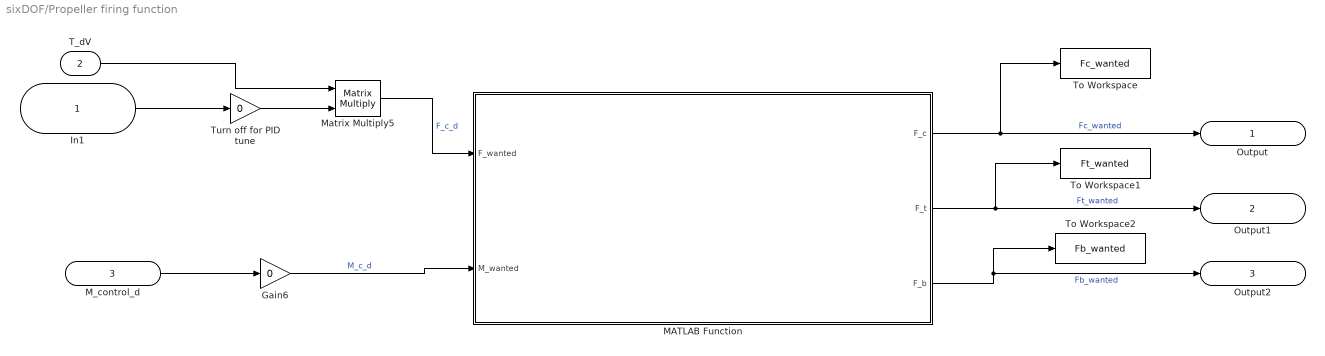
== system sixDOF/Propeller firing function ==
  In1 : Inport
  T_dV : Inport  Port=2
  M_control_d : Inport  Port=3
  Gain6 : Gain  Gain=0
  MATLAB Function : MATLAB Function  TreatAsAtomicUnit=on
  Matrix Multiply5 : Product  Multiplication=Matrix(*)
  To Workspace : ToWorkspace  VariableName=Fc_wanted  SaveFormat=Timeseries  SampleTime=-1
  To Workspace1 : ToWorkspace  VariableName=Ft_wanted  SaveFormat=Timeseries  SampleTime=-1
  To Workspace2 : ToWorkspace  VariableName=Fb_wanted  SaveFormat=Timeseries  SampleTime=-1
  Turn off for PID tune : Gain  Gain=0
  Output : Outport
  Output1 : Outport  Port=2
  Output2 : Outport  Port=3
  wires:
  Turn off for PID tune/1 -> Matrix Multiply5/2
  In1/1 -> Turn off for PID tune/1
  Matrix Multiply5/1 -> MATLAB Function/1(F_wanted)  "F_c_d"
  T_dV/1 -> Matrix Multiply5/1
  M_control_d/1 -> Gain6/1
  Gain6/1 -> MATLAB Function/2(M_wanted)  "M_c_d"
  MATLAB Function/2(F_t) -> To Workspace1/1, Output1/1  "Ft_wanted"
  MATLAB Function/3(F_b) -> Output2/1, To Workspace2/1  "Fb_wanted"
  MATLAB Function/1(F_c) -> To Workspace/1, Output/1  "Fc_wanted"

== system sixDOF/Trajectory Generation System <TBD> ==
  Constant : Constant  Value=[0;0;0]
  Constant4 : Constant  Value=[0.1; 0.2; 0.05]
  input trajectory^V : Outport
  theta_desired^V : Outport  Port=2
  wires:
  Constant4/1 -> theta_desired^V/1  "theta_desired^V"
  Constant/1 -> input trajectory^V/1  "input trajectory^V"

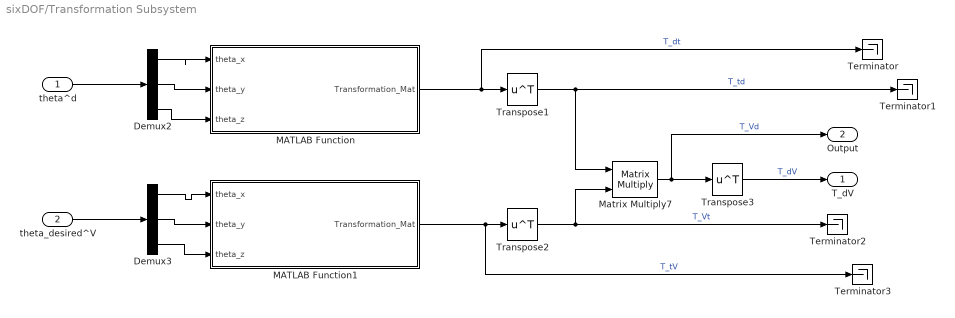
== system sixDOF/Transformation Subsystem ==
  theta^d : Inport
  theta_desired^V : Inport  Port=2
  Demux2 : Demux  Outputs=3
  Demux3 : Demux  Outputs=3
  MATLAB Function : MATLAB Function  TreatAsAtomicUnit=on
  MATLAB Function1 : MATLAB Function  TreatAsAtomicUnit=on
  Matrix Multiply7 : Product  Multiplication=Matrix(*)
  Terminator{,1..3} (4 alike) : Terminator
  Transpose1 : Math  Operator=transpose  SaturateOnIntegerOverflow=on
  Transpose2 : Math  Operator=transpose  SaturateOnIntegerOverflow=on
  Transpose3 : Math  Operator=transpose  SaturateOnIntegerOverflow=on
  T_dV : Outport
  Output : Outport  Port=2
  wires:
  Demux3/1 -> MATLAB Function1/1(theta_x)
  Demux2/1 -> MATLAB Function/1(theta_x)
  Transpose2/1 -> Terminator2/1, Matrix Multiply7/2  "T_Vt"
  Demux2/2 -> MATLAB Function/2(theta_y)
  MATLAB Function/1(Transformation_Mat) -> Terminator/1, Transpose1/1  "T_dt"
  Transpose1/1 -> Terminator1/1, Matrix Multiply7/1  "T_td"
  Demux2/3 -> MATLAB Function/3(theta_z)
  MATLAB Function1/1(Transformation_Mat) -> Terminator3/1, Transpose2/1  "T_tV"
  Matrix Multiply7/1 -> Output/1, Transpose3/1  "T_Vd"
  theta_desired^V/1 -> Demux3/1
  Demux3/3 -> MATLAB Function1/3(theta_z)
  Demux3/2 -> MATLAB Function1/2(theta_y)
  Transpose3/1 -> T_dV/1  "T_dV"
  theta^d/1 -> Demux2/1

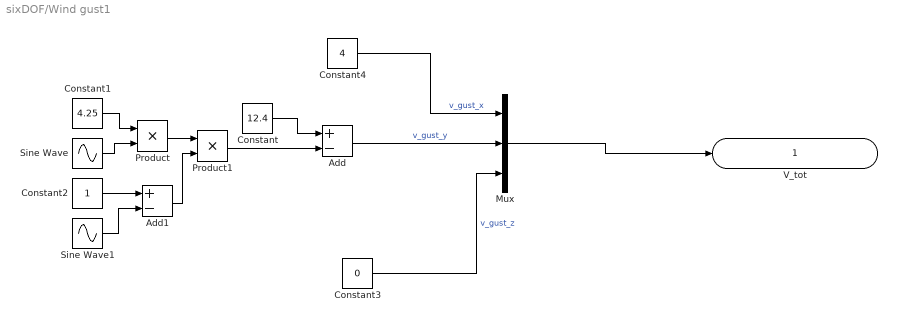
== system sixDOF/Wind gust1 ==
  Add : Sum  Inputs=+-
  Add1 : Sum  Inputs=+-
  Constant : Constant  Value=12.4
  Constant1 : Constant  Value=4.25
  Constant2 : Constant
  Constant3 : Constant  Value=0
  Constant4 : Constant  Value=4  VectorParams1D=off
  Mux : Mux  Inputs=3
  Product : Product
  Product1 : Product
  Sine Wave : Sin  Frequency=3*pi/T  SampleTime=0
  Sine Wave1 : Sin  Frequency=2*pi/T  Phase=pi/2  SampleTime=0
  V_tot : Outport
  wires:
  Constant/1 -> Add/1
  Constant1/1 -> Product/1
  Sine Wave/1 -> Product/2
  Constant2/1 -> Add1/1
  Sine Wave1/1 -> Add1/2
  Product/1 -> Product1/1
  Add1/1 -> Product1/2
  Product1/1 -> Add/2
  Add/1 -> Mux/2  "v_gust_y"
  Constant3/1 -> Mux/3  "v_gust_z"
  Mux/1 -> V_tot/1
  Constant4/1 -> Mux/1  "v_gust_x"

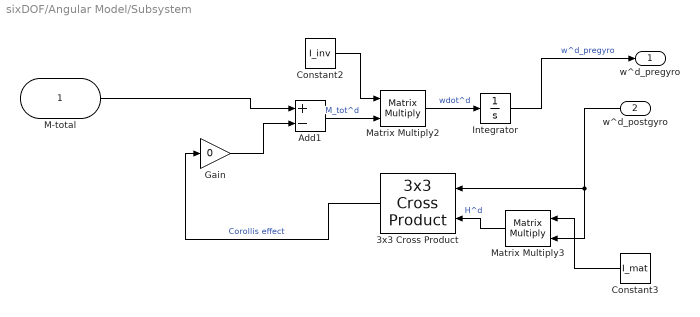
== system sixDOF/Angular Model/Subsystem ==
  M-total : Inport
  w^d_postgyro : Inport  Port=2
  3x3 Cross Product : sharedutil/3x3 Cross Product  aMode=aMode
      settings: SourceProductBaseCode=AE,PW,MT,UV,VE,VP
  Add1 : Sum  Inputs=+-
  Constant2 : Constant  Value=I_inv
  Constant3 : Constant  Value=I_mat
  Gain : Gain  Gain=0
  Integrator : Integrator  InitialCondition=[0;0;0]
  Matrix Multiply2 : Product  Multiplication=Matrix(*)
  Matrix Multiply3 : Product  Multiplication=Matrix(*)
  w^d_pregyro : Outport
  wires:
  Matrix Multiply3/1 -> 3x3 Cross Product/2  "H^d"
  Constant3/1 -> Matrix Multiply3/1
  Matrix Multiply2/1 -> Integrator/1  "wdot^d"
  w^d_postgyro/1 -> Matrix Multiply3/2, 3x3 Cross Product/1
  Constant2/1 -> Matrix Multiply2/1
  3x3 Cross Product/1 -> Gain/1  "Corollis effect"
  Add1/1 -> Matrix Multiply2/2  "M_tot^d"
  M-total/1 -> Add1/1
  Integrator/1 -> w^d_pregyro/1  "w^d_pregyro"
  Gain/1 -> Add1/2

== matlab function sixDOF/Transformation Subsystem/MATLAB Function ==
  data: theta_x input; Transformation_Mat output; theta_y input; theta_z input
function Transformation_Mat  = Euler(theta_x, theta_y, theta_z)

a = cos(theta_x)*cos(theta_z);
b = cos(theta_x)*sin(theta_z);
c = - sin(theta_x);
d = sin(theta_y)*sin(theta_x)*cos(theta_z) - cos(theta_y)*sin(theta_z);
e = sin(theta_y)*sin(theta_x)*sin(theta_z) + cos(theta_y)*cos(theta_z);
f = sin(theta_y)*cos(theta_x);
g = cos(theta_y)*sin(theta_x)*cos(theta_z) + sin(theta_y)*sin(theta_z);
h = cos(theta_y)*sin(theta_x)*sin(theta_z) - sin(theta_y)*cos(theta_z);
i = cos(theta_y)*cos(theta_x);

Transformation_Mat = [a b c;
    d e f;
    g h i];


end

== matlab function sixDOF/Gyroscope Model/MATLAB Function ==
  data: angvel input; gyroData output; acc input
function gyroData  = gyroscope(angvel, acc)
    % Ouputs: Angular velocity
    % Create gyroscope sensor object
    params = gyroparams         
    
    % Parameters for simulated signal
    N = 1;       % Number of samples
    Fs = 100;       % Sampling rate
    Fc = 0.25;      % Sinusoidal frequency
    
    % Create arrays
    t = (0:(1/Fs):((N-1)/Fs)).';
    acc = acc;          % Input accelerations
    angvel = angvel;
    %angvel(:,1) = 8*sin(2*pi*Fc*t);
    
    % Generate gyroscopic data
    imu = imuSensor('SampleRate', Fs, 'Gyroscope', params);
    imu.Gyroscope.MeasurementRange = 6.5;   % Maximum angular velocity gyroscope can measure
    imu.Gyroscope.Resolution = 1/Fs;           % Step size of digital measurements
    
    % Biases
    
    imu.Gyroscope.BiasInstability = 0.12 * 3.14159 / 180;       % rad/hr
    imu.Gyroscope.NoiseDensity = 0.15 * 3.14159 / 180;          % rad/s
    imu.Gyroscope.RandomWalk = 0.017 * 3.14159 / 180;           % rad/sqrt(hr)
    imu.Gyroscope.TemperatureBias = 0.25 * 3.14159 / 180;       % rad/s
    imu.Gyroscope.AccelerationBias = 0.3;
    
    % Define real accelerations
    %acc(:,1) = 1;
    [~, gyroData] = imu(acc, angvel);

end

== matlab function sixDOF/Transformation Subsystem/MATLAB Function1 ==
  data: theta_x input; Transformation_Mat output; theta_y input; theta_z input
function Transformation_Mat  = Euler(theta_x, theta_y, theta_z)

a = cos(theta_x)*cos(theta_z);
b = cos(theta_x)*sin(theta_z);
c = - sin(theta_x);
d = sin(theta_y)*sin(theta_x)*cos(theta_z) - cos(theta_y)*sin(theta_z);
e = sin(theta_y)*sin(theta_x)*sin(theta_z) + cos(theta_y)*cos(theta_z);
f = sin(theta_y)*cos(theta_x);
g = cos(theta_y)*sin(theta_x)*cos(theta_z) + sin(theta_y)*sin(theta_z);
h = cos(theta_y)*sin(theta_x)*sin(theta_z) - sin(theta_y)*cos(theta_z);
i = cos(theta_y)*cos(theta_x);

Transformation_Mat = [a b c;
    d e f;
    g h i];


end

== matlab function sixDOF/Propeller firing function/MATLAB Function ==
  data: F_wanted input; F_c output; M_wanted input; F_t output; F_b output
function [F_c, F_t, F_b] = propeller_required_forces_control(F_wanted, M_wanted)

%% Load propeller arms data
prop_arms;


%% Decompose force and moment input

F_x = F_wanted(1);
F_y = F_wanted(2);
F_z = F_wanted(3);

M_x = M_wanted(1);
M_y = M_wanted(2);
M_z = M_wanted(3);

%% Find control forces

F_c3 = 2*(M_x + M_y + F_y)/(-yc_1 + zc_1 - yc_2 + zc_2 - 2*yc_3 + 2*zc_3);
F_c2 = F_c3/2;
F_c1 = F_c2;

%% Find top and bottom forces

F_t1 = 1/10 * F_z + M_y/6*(xt_1 + xt_2 + xt_3 + xt_4 + xb_1 + xb_2 + xb_5 + xb_6);
F_t2 = F_t1;
F_t3 = F_t1;
F_t4 = F_t1;
F_b1 = F_t1;
F_b2 = F_t1;
F_b5 = F_t1;
F_b6 = F_t1;

F_b3 = 1/10 * F_z;
F_b4 = F_b3;


%% Make matrix
F_c = [F_c1; F_c2; Fc3];
F_t = [F_t1; F_t2; F_t3; F_t4];
F_b = [F_b1; F_b2; F_b3; F_b4; F_b5; F_b6];

end

== matlab function sixDOF/Accelerometer Model/Input in the disturbance frame ==
  data: angvel input; accelData output; acc input
function accelData  = accelerometer(angvel, acc)
    %% Outputs: translational acceleration
    %
    % Create gyroscope sensor object
    params = accelparams 
    
    % Parameters for simulated signal
    N = 1;       % Number of samples
    Fs = 100;       % Sampling rate
    Fc = 0.25;      % Sinusoidal frequency
    
    
    % Create arrays
    t = (0:(1/Fs):((N-1)/Fs)).';
    acc = acc;          %Input accelerations
    orient = quaternion.ones(N, 1);
    angvel = angvel;
    
    % Generate acceleration data
    imu = imuSensor('SampleRate', Fs, 'Accelerometer', params);
    imu.Accelerometer.MeasurementRange = 10;   % Maximum acceleration accelerometer can measure
    imu.Accelerometer.Resolution = 1/Fs;           % Step size of digital measurements
    
    % Biases
    imu.Accelerometer.BiasInstability = 7.5 / 1000;
    imu.Accelerometer.NoiseDensity = 150 / 1000 / 1000;
    imu.Accelerometer.TemperatureBias = 50 / 1000 / 1000;
    
    
    imu = imuSensor('SampleRate', Fs, 'Accelerometer', params);
    
    accelData = imu(acc, angvel, orient);

end
